simulink model "modelo_lqr"  (R2023a)
settings: Solver=ode45  StartTime=0.0  StopTime=10.0  MaxStep=0.01  RelTol=1e-3
model workspace: external: MATLAB File C:\Users\pinki\OneDrive\aviãozinho\monociclo\numvars.m (data not in the file)
values from neighbouring files (symbols this model uses):
  Ard = [Ar(1,1) Ar(1,3:end) ... (first row only)    [Modelo_mono.m]    (also in workspace.mat = [0 0 -31.2551437046 31.2551437046 0 0 0 0 0 0 -92.3888975157)
  Brd = [Br(1,:) ... (first row only)    [Modelo_mono.m]    (also in workspace.mat = [0  0; 0  0; 50297.8358889  0; -78.116759971  0; 0  238.3657)
  Crd = [1 0 0 0 0 0 0 1 0 0 0 0 ... (36 elements, 6x6)]    [workspace.mat]
  Jbw = 0.07689    [gab_numvars.m]    (also in modelo.mat; numvars.m; workspace.mat = 0.026534412)
  Jr = 0.013472    [gab_numvars.m]    (also in modelo.mat; numvars.m; workspace.mat = 0.0001347355)
  K = lqr(Ard,Brd,Qc,Rc)    [Modelo_mono.m]    (also in cascatinha_v3.m = [tprK,0; workspace.mat = [-891.058429104  -1.00065730536e-12  -0.217264538579  -159.5)
  pos0 = [0.05; 0.1; 0.004; 0.07]    [numvars.m]
undefined symbols (not defined in the file or in its folder): Drd
settings Model: Creator=pinki  LastModifiedBy=pinki
settings DataIOCC: InspectSignalLogs=on

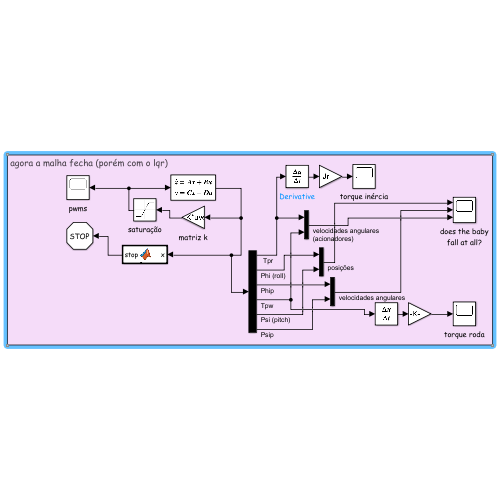
[thumbnail: Simulink's stored preview of the top-level diagram]
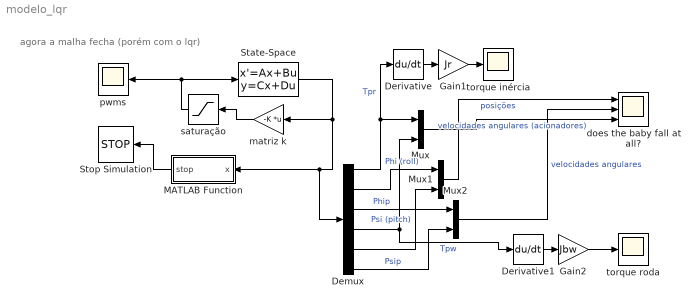
== system modelo_lqr ==
  note: agora a malha fecha (porém com o lqr)
  Demux : Demux  Outputs=6
  Derivative : Derivative
  Derivative1 : Derivative
  Gain1 : Gain  Gain=Jr
  Gain2 : Gain  Gain=Jbw
  MATLAB Function : MATLAB Function  TreatAsAtomicUnit=on
  Mux : Mux  Inputs=2
  Mux1 : Mux  Inputs=2
  Mux2 : Mux  Inputs=2
  State-Space : StateSpace  A=Ard  B=Brd  C=Crd  D=Drd  InitialCondition=pos0  ParameterTunability=Unconstrained
  Stop Simulation : Stop
  does the baby fall at all? : Scope  NumInputPorts=3
  matriz k : Gain  Gain=-K  Multiplication=Matrix(K*u) (u vector)
  pwms : Scope
  saturação : Saturate  UpperLimit=1  LowerLimit=-1
  torque inércia : Scope
  torque roda : Scope
  wires:
  matriz k/1 -> saturação/1
  State-Space/1 -> Demux/1, MATLAB Function/1(x), matriz k/1
  Demux/1 -> Derivative/1, Mux/1  "Tpr"
  Demux/4 -> Mux/2, Derivative1/1  "Tpw"
  Demux/3 -> Mux2/1  "Phip"
  saturação/1 -> pwms/1, State-Space/1
  MATLAB Function/1(stop) -> Stop Simulation/1
  Derivative/1 -> Gain1/1
  Gain1/1 -> torque inércia/1
  Derivative1/1 -> Gain2/1
  Gain2/1 -> torque roda/1
  Demux/2 -> Mux1/1  "Phi (roll)"
  Demux/6 -> Mux2/2  "Psip"
  Demux/5 -> Mux1/2  "Psi (pitch)"
  Mux1/1 -> does the baby fall at all?/1  "posições"
  Mux2/1 -> does the baby fall at all?/2  "velocidades angulares"
  Mux/1 -> does the baby fall at all?/3  "velocidades angulares (acionadores)"

== matlab function modelo_lqr/MATLAB Function ==
  data: x input; stop output
function stop = fcn(x)

Roll = x(2);
Pitch = x(5);

%% assumindo deslocamento m'aximo de 30 graus ou 0,5 rad...
limite = 0.5;

stop = abs(Pitch)>limite || abs(Roll)>limite;
